simulink library "cstextras"  (R2025b)
settings: Solver=ode45  StartTime=0.0  StopTime=10.0  RelTol=1e-3
values from neighbouring files (symbols this model uses):
  D = ltipack.lftdataFRD(IC,ltipack.LFTBlockWrapper(blk))    [ControlDesignBlock.m]    (also in DynamicBlock.m = pidstd(ltipack_ssdata(blk)); delayss.m = ltipack.ssdata(a0,b,c,[d0 q;s zeros(length(tau))],[],Ts))
  P = randp_(blk,varargin{:})    [tunableBlock.m]
libraries: $bdroot x1
settings Model: FPTRunName=Active  Creator=The MathWorks, Inc.  LastModifiedBy=The MathWorks, Inc.
settings SolverCC: AlgebraicLoopSolver=TrustRegion  MaxZcPerStep=1.0
settings DataIOCC: LimitDataPoints=on  SaveFormat=Array  SignalLoggingSaveFormat=ModelDataLogs  ReturnWorkspaceOutputs=off
settings OptimizationCC: BlockReduction=off  BooleanDataType=off  ExpressionDepthLimit=2147483647.0  LifeSpan=inf
settings DebuggingCC: SaveWithParameterizedLinksMsg=none  UnderspecifiedInitializationDetection=Classic  MergeDetectMultiDrivingBlocksExec=none  SignalResolutionControl=TryResolveAllWithWarning  FcnCallInpInsideContextMsg=warning  UnconnectedInputMsg=warning  UnconnectedOutputMsg=warning  UnconnectedLineMsg=warning  AllowSymbolicDim=off  StateNameClashWarn=warning  SubsystemReferenceDiagnosticForUnitTest=warning  SFUnexpectedBacktrackingDiag=warning  SFNoUnconditionalDefaultTransitionDiag=warning  SFExecutionAtInitializationDiag=none  ArithmeticOperatorsInVariantConditions=warning
settings HardwareCC: ProdBitPerPointer=32.0  ProdBitPerSizeT=32.0  ProdBitPerPtrDiffT=32.0  ProdLargestAtomicFloat=None  ProdIntDivRoundTo=Undefined  ProdEndianess=Unspecified  ProdWordSize=32.0  ProdHWDeviceType=32-bit Generic  TargetUnknown=on
settings ModelReferenceCC: EnableRefExpFcnMdlSchedulingChecks=on  PropagateSignalLabelsOutOfModel=off
settings SFSimCC: SimUseLocalCustomCode=off
settings RTWCC: RTWUseLocalCustomCode=off  GPUComputeCapability=3.5  DLArmComputeVersion=19.05  LargeConstantGeneration=WriteOnlyDNNConstantsToDataFiles
settings CodeAppCC: StateflowObjectComments=on
settings GRTTargetCC: TargetLangStandard=C89/C90 (ANSI)  CombineOutputUpdateFcns=off  GRTInterface=on
settings ConfigComp: CovMetricSettings=dw  CovSaveCumulativeToWorkspaceVar=on  CovSaveSingleToWorkspaceVar=on  CovExternalEMLEnable=off  CovSFcnEnable=off

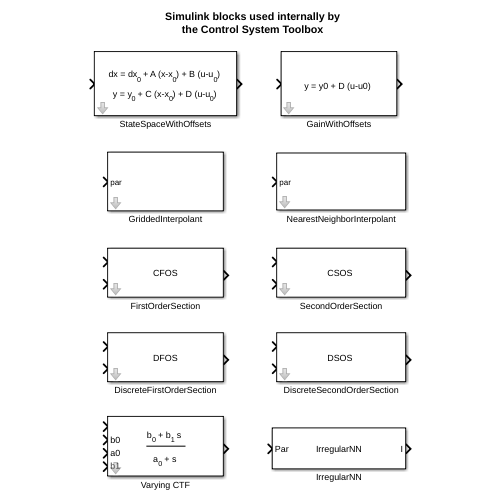
[thumbnail: Simulink's stored preview of the top-level diagram]
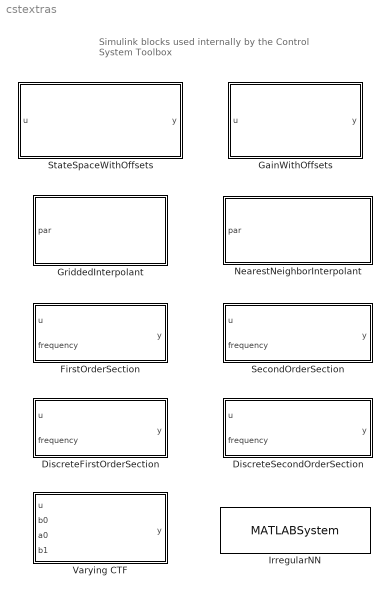
== system cstextras ==
  note: Simulink blocks used internally by
      | the Control System Toolbox
  DiscreteFirstOrderSection : Subsystem  VariantControl=(default)  mask(DiscreteFirstOrderSection){Ts=1, w0=0}
      mask prompts: Ts "Sample time Ts"; w0 "Pre-warping frequency w0"
      mask help:
      | Implements the Tustin discretization of the first-order lowpass filter
      |
      |               w
      | F(s) = ---------
      |            s + w
      |
      | where w is the cutoff frequency value fed to the "frequency" port. The discrete transfer function is obtained by Tustin transformation with pre-warping at the frequency w0. The default value w0=0 corresponds to the usual bilinear transformation:
      |
      | s = 2/Ts (z-1)/(z+1).
      mask init:
      | if w0>0
      |    tau = tan(w0*Ts/2)/w0;
      | else
      |    tau = Ts/2;
      | end
      mask Display: text(0.4,0.5,'DFOS')
  DiscreteSecondOrderSection : Subsystem  VariantControl=order2  mask(DiscreteSecondOrderSection){zeta=0.7, Ts=1, w0=0}
      mask prompts: zeta "Damping ratio"; Ts "Sample time Ts"; w0 "Pre-warping frequency w0"
      mask help:
      | Implements the Tustin discretization of the second-order lowpass filter
      |
      |                          w^2
      | F(s) = ---------------------------------------
      |            s^2 + 2 * zeta * w * s + w^2
      |
      | where zeta is the damping ratio and w is the cutoff frequency value fed to the "frequency" port. The discrete transfer function is obtained by Tustin transformation with pre-warping at the frequency w0. The default value w0=0 corresponds to the usual bilinear transformation:
      |
      | s = 2/Ts (z-1)/(z+1).
      mask init:
      | if w0>0
      |    tau = tan(w0*Ts/2)/w0;
      | else
      |    tau = Ts/2;
      | end
      mask Display: text(0.4,0.5,'DSOS')
  FirstOrderSection : Subsystem  VariantControl=(default)  mask(FirstOrderSection){}
      mask help:
      | Implements the analog first-order lowpass filter
      |
      |               w
      | F(s) = ---------
      |            s + w
      |
      | where w is the cutoff frequency value fed to the "frequency" port.
      mask Display: text(0.4,0.5,'CFOS')
  GainWithOffsets : Subsystem  mask{D=0, u0=0, y0=0}
      mask prompts: D "Control:simulink:LPVMask34"; u0 "Control:simulink:LPVMask8"; y0 "Control:simulink:LPVMask9"
      mask help: Control:simulink:SSOffsets2
      mask Help: eval('helpview(''control'',''VaryingSSCT'');')
      mask DialogControl D Prompt: D matrix:
      mask DialogControl u0 Prompt: Input offset:
      mask DialogControl y0 Prompt: Output offset:
      mask Display: text(0.5,0.5,'y = y0 + D (u-u0)','horizontalAlignment', 'center','texmode','on')
  GriddedInterpolant : Subsystem  mask{Table=[], INFO=[], IndexSearch=Binary search, IndexBegin=on}
      mask prompts: Table "Vectorized data"; INFO "Structural info"; IndexSearch "Control:simulink:LPVMask25"; IndexBegin "Control:simulink:LPVMask26"
      mask help: Control:simulink:GriddedInterp1
      mask init:
      | if controllib.internal.blocks.safeMaskUpdate(gcb)
      |    controllib.internal.blocks.lpv.GriddedInterpolantMask(gcb,Table,INFO,IndexSearch,IndexBegin);
      | end
      mask TypeOptions IndexSearch: Binary search | Linear search
      mask DialogControl IndexSearch Prompt: Index search method:
      mask DialogControl IndexBegin Prompt: Begin index search using previous index result
  IrregularNN : MATLABSystem  System=controllib.internal.blocks.lpv.IrregularNN  d=2  BP=[ (1:10)', (0:9)'*10 ]  SimulateUsing=Interpreted execution
      mask Type: controllib.internal.blocks.lpv.IrregularNN
  NearestNeighborInterpolant : Subsystem  mask{Table=[], INFO=[]}
      mask prompts: Table "Vectorized data"; INFO "Structural info"
      mask init:
      | if controllib.internal.blocks.safeMaskUpdate(gcb)
      |     controllib.internal.blocks.lpv.NNInterpolantMask(gcb,Table,INFO);
      | end
  SecondOrderSection : Subsystem  VariantControl=order2  mask(SecondOrderSection){zeta=1}
      mask prompts: zeta "Damping ratio"
      mask help:
      | Implements the analog second-order lowpass filter
      |
      |                          w^2
      | F(s) = ---------------------------------------
      |            s^2 + 2 * zeta * w * s + w^2
      |
      | where zeta is the damping ratio and w is the cutoff frequency value fed to the "frequency" port.
      mask Display: text(0.4,0.5,'CSOS')
  StateSpaceWithOffsets : Subsystem  mask{A=0, B=0, C=0, D=0, IC=0, Ts=0, dx0=0, x0=0, u0=0, y0=0}
      mask prompts: A "Control:simulink:LPVMask31"; B "Control:simulink:LPVMask32"; C "Control:simulink:LPVMask33"; D "Control:simulink:LPVMask34"; IC "Control:simulink:LPVMask13"; Ts "Control:simulink:VaryingTFLabel2"; dx0 "Control:simulink:LPVMask11a"; x0 "Control:simulink:LPVMask10"; u0 "Control:simulink:LPVMask8"; y0 "Control:simulink:LPVMask9"
      mask help: Control:simulink:SSOffsets1
      mask init:
      | IC = IC(:);
      | if controllib.internal.blocks.safeMaskUpdate(gcb)
      |     REAL = isreal(A) && isreal(B) && isreal(C) && isreal(D) && ...
      |         isreal(dx0) && isreal(x0) && isreal(u0) && isreal(y0) && isreal(IC);
      |     controllib.internal.blocks.lti.StateSpaceWithOffsetMask(gcb,Ts,REAL)
      | end
      mask Help: eval('helpview(''control'',''VaryingSSCT'');')
      mask DialogControl Container4 Prompt: Control:simulink:SSOffsets3
      mask DialogControl A Prompt: A matrix:
      mask DialogControl B Prompt: B matrix:
      mask DialogControl C Prompt: C matrix:
      mask DialogControl D Prompt: D matrix:
      mask DialogControl Ts Prompt: Sample time (-1 for inherited):
      mask DialogControl Container5 Prompt: Control:simulink:VaryingSSLabel8
      mask DialogControl dx0 Prompt: State derivative/update offset:
      mask DialogControl x0 Prompt: State offset:
      mask DialogControl u0 Prompt: Input offset:
      mask DialogControl y0 Prompt: Output offset:
      mask Display:
      | [eqx,eqy] = controllib.internal.blocks.varying.varyingSS_icon((Ts==0),true,true,true,true,true);
      | text(0.5,0.65,eqx,'horizontalAlignment', 'center','texmode','on')
      | text(0.5,0.35,eqy,'horizontalAlignment', 'center','texmode','on')
  Varying CTF : Subsystem  mask(Varying Transfer Function){N=1}
      mask prompts: N "Control:simulink:VaryingTFLabel1"
      mask help: Control:simulink:VaryingTF1OLD
      mask init:
      | if N~=round(N)
      |    hCB = get_param(gcb,'handle');
      |    DAStudio.slerror('Control:simulink:InvalidOrder',hCB)
      | end
      | SimStatus = get_param(bdroot,'SimulationStatus');
      | if any(strcmp(SimStatus,{'initializing','updating','stopped'}))
      |    controllib.internal.blocks.varying.varyingCTF(gcb,N)
      | end
      mask Help: eval('ctrlguihelp(''VaryingTFCT_OLD'');')
      mask DialogControl N Prompt: Transfer function order:
      mask Display:
      | port_label('input',2,'b0');
      | port_label('input',4,'b1');
      | port_label('input',3,'a0');
      | plot([0.325 0.675],[0.5 0.5])
      | text(0.5, 0.7, 'b_0 + b_1 s' ,...
      |         'horizontalAlignment', 'center','texmode','on')
      | text(0.5, 0.3, 'a_0 + s' ,...
      |         'horizontalAlignment', 'center','texmode','on')

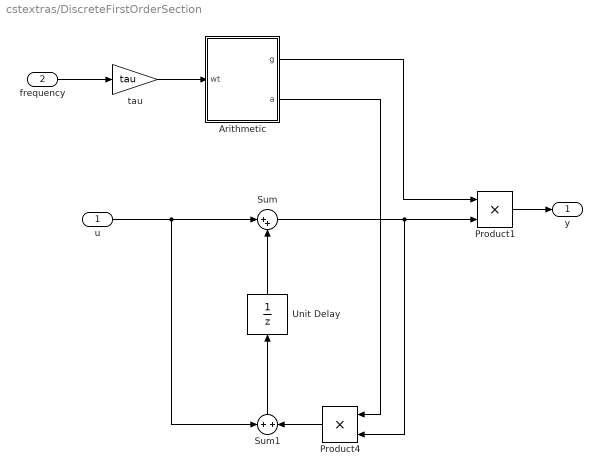
== system cstextras/DiscreteFirstOrderSection ==
  u : Inport
  frequency : Inport  Port=2
  Arithmetic : Subsystem
  Product1 : Product
  Product4 : Product
  Sum : Sum  Inputs=|++
  Sum1 : Sum  Inputs=+|+
  Unit Delay : UnitDelay  SampleTime=Ts  HasFrameUpgradeWarning=on
  tau : Gain  Tag=#GainSurfaceTarget_  Gain=tau
  y : Outport  VectorParamsAs1DForOutWhenUnconnected=off
  wires:
  u/1 -> Sum1/1, Sum/1
  Unit Delay/1 -> Sum/2
  Sum1/1 -> Unit Delay/1
  Product4/1 -> Sum1/2
  Sum/1 -> Product1/2, Product4/2
  Product1/1 -> y/1
  frequency/1 -> tau/1
  Arithmetic/1(g) -> Product1/1
  Arithmetic/2(a) -> Product4/1
  tau/1 -> Arithmetic/1(wt)

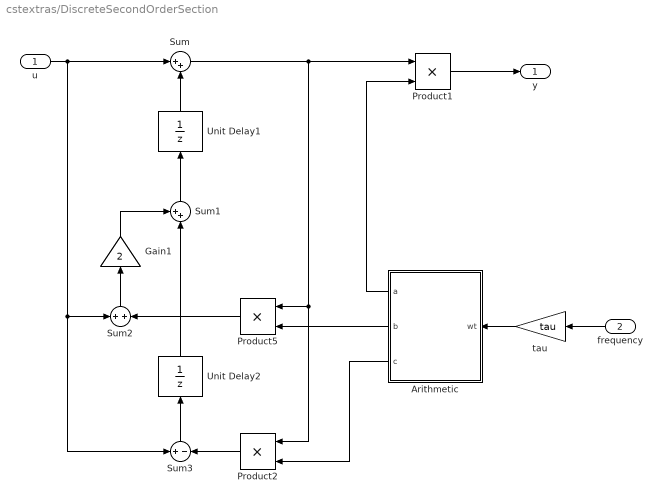
== system cstextras/DiscreteSecondOrderSection ==
  u : Inport
  frequency : Inport  Port=2
  Arithmetic : Subsystem
  Gain1 : Gain  Gain=2
  Product1 : Product
  Product2 : Product
  Product5 : Product
  Sum : Sum  Inputs=|++
  Sum1 : Sum  Inputs=++|
  Sum2 : Sum  Inputs=+|+
  Sum3 : Sum  Inputs=+|-
  Unit Delay1 : UnitDelay  SampleTime=Ts  HasFrameUpgradeWarning=on
  Unit Delay2 : UnitDelay  SampleTime=Ts  HasFrameUpgradeWarning=on
  tau : Gain  Tag=#GainSurfaceTarget_  Gain=tau
  y : Outport  VectorParamsAs1DForOutWhenUnconnected=off
  wires:
  u/1 -> Sum3/1, Sum2/1, Sum/1
  Unit Delay1/1 -> Sum/2
  Sum1/1 -> Unit Delay1/1
  Gain1/1 -> Sum1/1
  Sum2/1 -> Gain1/1
  Unit Delay2/1 -> Sum1/2
  Product5/1 -> Sum2/2
  Sum/1 -> Product1/1, Product5/1, Product2/1
  Product1/1 -> y/1
  Sum3/1 -> Unit Delay2/1
  Product2/1 -> Sum3/2
  Arithmetic/1(a) -> Product1/2
  Arithmetic/2(b) -> Product5/2
  Arithmetic/3(c) -> Product2/2
  frequency/1 -> tau/1
  tau/1 -> Arithmetic/1(wt)

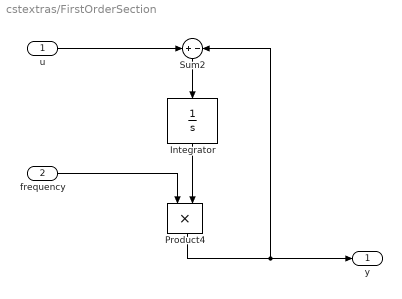
== system cstextras/FirstOrderSection ==
  u : Inport
  frequency : Inport  Port=2
  Integrator : Integrator
  Product4 : Product
  Sum2 : Sum  Inputs=+|-
  y : Outport  VectorParamsAs1DForOutWhenUnconnected=off
  wires:
  Product4/1 -> Sum2/2, y/1
  Sum2/1 -> Integrator/1
  frequency/1 -> Product4/1
  Integrator/1 -> Product4/2
  u/1 -> Sum2/1

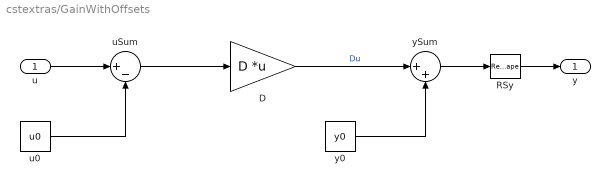
== system cstextras/GainWithOffsets ==
  u : Inport
  D : Gain  Gain=D  Multiplication=Matrix(K*u)
  RSy : Reshape
  u0 : Constant  Value=u0
  uSum : Sum  Inputs=|+-
  y0 : Constant  Value=y0
  ySum : Sum  Inputs=|++
  y : Outport  VectorParamsAs1DForOutWhenUnconnected=off
  wires:
  RSy/1 -> y/1
  ySum/1 -> RSy/1
  D/1 -> ySum/1  "Du"
  uSum/1 -> D/1
  y0/1 -> ySum/2
  u/1 -> uSum/1
  u0/1 -> uSum/2

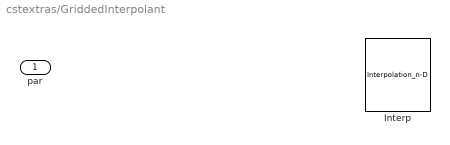
== system cstextras/GriddedInterpolant ==
  par : Inport
  Interp : Interpolation_n-D  NumberOfTableDimensions=1  Table=Table  InternalRulePriority=Speed
      settings: InputPortMap=u0,u1

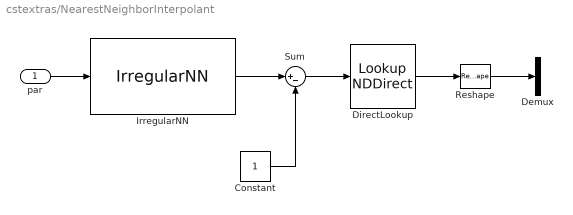
== system cstextras/NearestNeighborInterpolant ==
  par : Inport
  Constant : Constant
  Demux : Demux  Outputs=2
  DirectLookup : LookupNDDirect  InputsSelectThisObjectFromTable=Vector  Table=[]  DiagnosticForOutOfRangeInput=None
  IrregularNN : $bdroot/IrregularNN  d=2  BP=cat(2,P{:})  SimulateUsing=Interpreted execution
  Reshape : Reshape  OutputDimensionality=Column vector (2-D)
  Sum : Sum  Inputs=|+-
  wires:
  par/1 -> IrregularNN/1
  IrregularNN/1 -> Sum/1
  Sum/1 -> DirectLookup/1
  Constant/1 -> Sum/2
  DirectLookup/1 -> Reshape/1
  Reshape/1 -> Demux/1

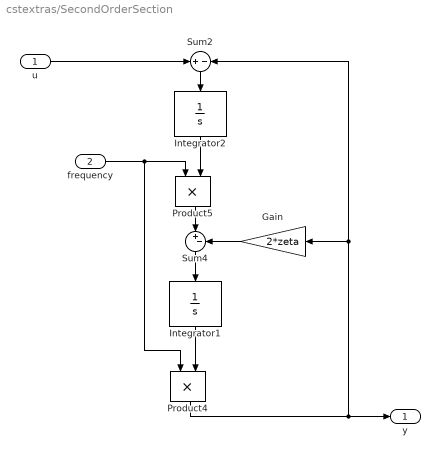
== system cstextras/SecondOrderSection ==
  u : Inport
  frequency : Inport  Port=2
  Gain : Gain  Gain=2*zeta
  Integrator1 : Integrator
  Integrator2 : Integrator
  Product4 : Product
  Product5 : Product
  Sum2 : Sum  Inputs=+|-
  Sum4 : Sum  Inputs=|+-
  y : Outport  VectorParamsAs1DForOutWhenUnconnected=off
  wires:
  Sum2/1 -> Integrator2/1
  Product4/1 -> Sum2/2, Gain/1, y/1
  Product5/1 -> Sum4/1
  Integrator1/1 -> Product4/2
  Sum4/1 -> Integrator1/1
  frequency/1 -> Product5/1, Product4/1
  u/1 -> Sum2/1
  Integrator2/1 -> Product5/2
  Gain/1 -> Sum4/2

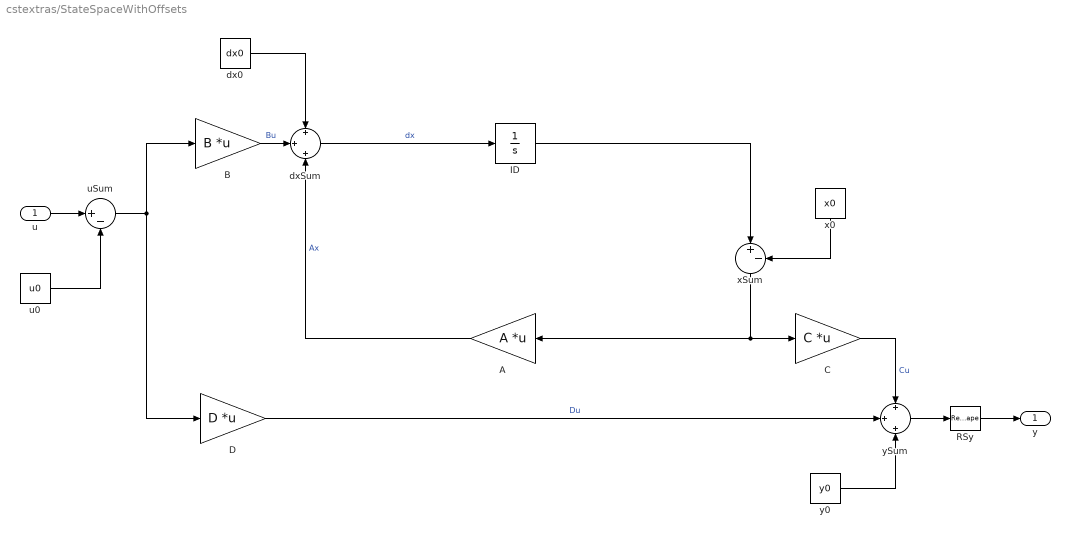
== system cstextras/StateSpaceWithOffsets ==
  u : Inport  SampleTime=Ts
  A : Gain  Gain=A  Multiplication=Matrix(K*u)
  B : Gain  Gain=B  Multiplication=Matrix(K*u)
  C : Gain  Gain=C  Multiplication=Matrix(K*u)
  D : Gain  Gain=D  Multiplication=Matrix(K*u)
  ID : Integrator  InitialCondition=IC
  RSy : Reshape
  dx0 : Constant  Value=dx0
  dxSum : Sum  Inputs=+|+|+
  u0 : Constant  Value=u0
  uSum : Sum  Inputs=|+-
  x0 : Constant  Value=x0
  xSum : Sum  Inputs=|+-
  y0 : Constant  Value=y0
  ySum : Sum  Inputs=+|+|+
  y : Outport  VectorParamsAs1DForOutWhenUnconnected=off
  wires:
  RSy/1 -> y/1
  ySum/1 -> RSy/1
  D/1 -> ySum/2  "Du"
  C/1 -> ySum/1  "Cu"
  uSum/1 -> D/1, B/1
  A/1 -> dxSum/3  "Ax"
  dx0/1 -> dxSum/1
  xSum/1 -> A/1, C/1
  B/1 -> dxSum/2  "Bu"
  y0/1 -> ySum/3
  u/1 -> uSum/1
  u0/1 -> uSum/2
  x0/1 -> xSum/2
  dxSum/1 -> ID/1  "dx"
  ID/1 -> xSum/1

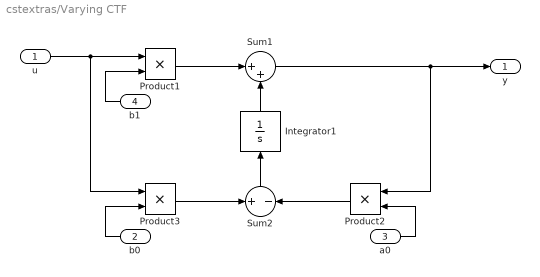
== system cstextras/Varying CTF ==
  u : Inport
  b0 : Inport  Port=2
  a0 : Inport  Port=3
  b1 : Inport  Port=4
  Integrator1 : Integrator
  Product1 : Product  InputSameDT=on  RndMeth=Zero  SaturateOnIntegerOverflow=on  OutDataTypeStr=Inherit: Same as first input
  Product2 : Product  InputSameDT=on  RndMeth=Zero  SaturateOnIntegerOverflow=on  OutDataTypeStr=Inherit: Same as first input
  Product3 : Product  InputSameDT=on  RndMeth=Zero  SaturateOnIntegerOverflow=on  OutDataTypeStr=Inherit: Same as first input
  Sum1 : Sum  Inputs=|++  InputSameDT=on  SaturateOnIntegerOverflow=on  OutDataTypeStr=Inherit: Same as first input
  Sum2 : Sum  Inputs=+|-  InputSameDT=on  SaturateOnIntegerOverflow=on  OutDataTypeStr=Inherit: Same as first input
  y : Outport  VectorParamsAs1DForOutWhenUnconnected=off
  wires:
  a0/1 -> Product2/2
  b0/1 -> Product3/2
  Product2/1 -> Sum2/2
  Product3/1 -> Sum2/1
  Sum2/1 -> Integrator1/1
  Integrator1/1 -> Sum1/2
  Sum1/1 -> Product2/1, y/1
  Product1/1 -> Sum1/1
  b1/1 -> Product1/2
  u/1 -> Product3/1, Product1/1

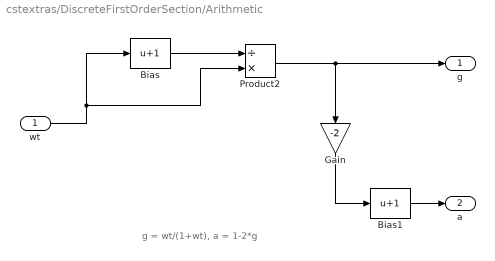
== system cstextras/DiscreteFirstOrderSection/Arithmetic ==
  note: g = wt/(1+wt), a = 1-2*g
  wt : Inport
  Bias : Bias  Bias=1  SaturateOnIntegerOverflow=off
  Bias1 : Bias  Bias=1  SaturateOnIntegerOverflow=off
  Gain : Gain  Gain=-2
  Product2 : Product  Inputs=/*
  g : Outport
  a : Outport  Port=2
  wires:
  Product2/1 -> g/1, Gain/1
  wt/1 -> Bias/1, Product2/2
  Gain/1 -> Bias1/1
  Bias/1 -> Product2/1
  Bias1/1 -> a/1

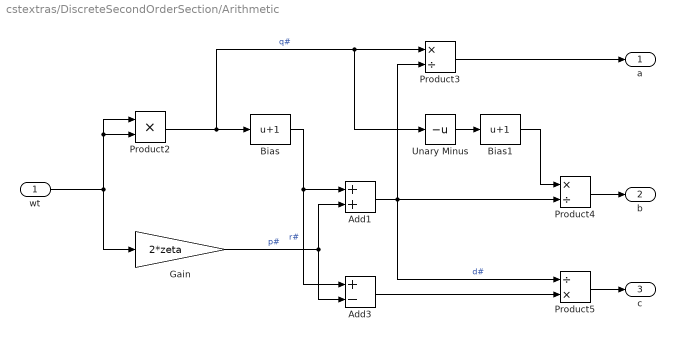
== system cstextras/DiscreteSecondOrderSection/Arithmetic ==
  wt : Inport
  Add1 : Sum
  Add3 : Sum  Inputs=+-
  Bias : Bias  Bias=1  SaturateOnIntegerOverflow=off
  Bias1 : Bias  Bias=1  SaturateOnIntegerOverflow=off
  Gain : Gain  Gain=2*zeta
  Product2 : Product
  Product3 : Product  Inputs=*/
  Product4 : Product  Inputs=*/
  Product5 : Product  Inputs=/*
  Unary Minus : UnaryMinus
  a : Outport
  b : Outport  Port=2
  c : Outport  Port=3
  wires:
  wt/1 -> Gain/1, Product2/2, Product2/1
  Product2/1 -> Bias/1, Unary Minus/1, Product3/1  "q#"
  Bias/1 -> Add3/1, Add1/1  "r#"
  Gain/1 -> Add1/2, Add3/2  "p#"
  Add1/1 -> Product5/1, Product4/2, Product3/2  "d#"
  Product3/1 -> a/1
  Bias1/1 -> Product4/1
  Product4/1 -> b/1
  Product5/1 -> c/1
  Add3/1 -> Product5/2
  Unary Minus/1 -> Bias1/1
